simulink model "gm_uz_ssi_interface_2023a"  (R2023a)
settings: Solver=FixedStepDiscrete  StartTime=0.0  StopTime=0.0025  RelTol=1e-3
undefined symbols (not defined in the file or in its folder): binary_or_gray, bit_sum, delay_first_clk_on_off, f_ADC, f_clock, PLL, ssi_clk_divider, ssi_encoder_bit_width_multi_turn, ssi_encoder_bit_width_single_turn, ssi_encoder_number_of_status_bits, t_ADC, t_clock
libraries: hdlmdlgenlib x111, hdlsllib x62, simulink x27, simulink_extras x7
(part 2 of 4)

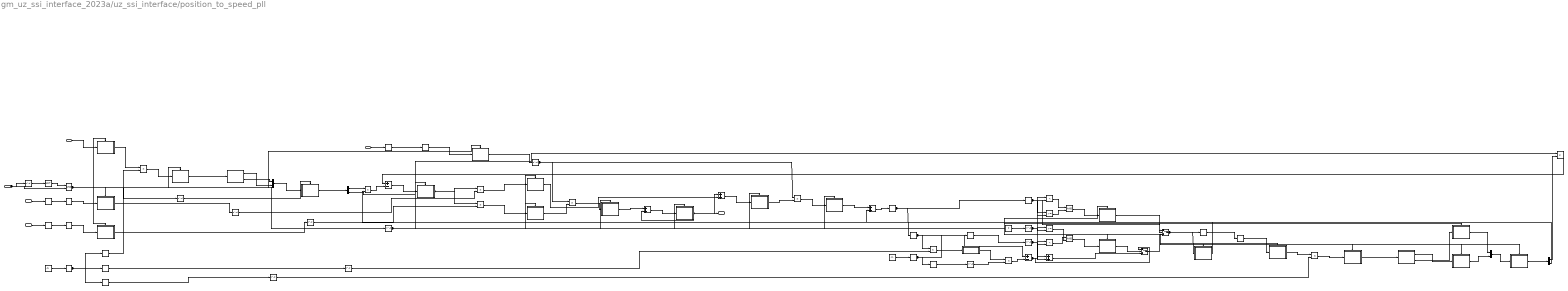
== system gm_uz_ssi_interface_2023a/uz_ssi_interface/position_to_speed_pll ==
  note: pi_controller
  note: +/- 198000
  note: -2 ... 2
  note: wrap 2pi
  note: <<1
  note: phase discriminator
  note: -1 ... 1
  note: pll
  note: -1 ... 1
  note: integrator
  note: 20
  note: +/- 1300
  note: remainder
  position_mech_SI : Inport  OutDataTypeStr=fixdt(0, 27, 24)  PortDimensions=1  SampleTime=1e-08
  t_sample : Inport  Port=2  OutDataTypeStr=fixdt(0, 18, 24)  PortDimensions=1  SampleTime=1e-08
  kp_pll : Inport  Port=3  OutDataTypeStr=fixdt(0, 18, 5)  PortDimensions=1  SampleTime=1e-08
  ki_pll : Inport  Port=4  OutDataTypeStr=fixdt(0, 18, 0)  PortDimensions=1  SampleTime=1e-08
  Trigger : Inport  Port=5  OutDataTypeStr=boolean  SampleTime=1e-08
  AND : Logic  AllPortsSameDT=off  OutDataTypeStr=boolean  SampleTime=1e-08
  AND1 : Logic  AllPortsSameDT=off  OutDataTypeStr=boolean  SampleTime=1e-08
  Constant1 : Constant  Value=0.1591548919677734375  OutDataTypeStr=fixdt(0, 18, 20)  SampleTime=1e-08
  Constant7 : Constant  Value=0  OutDataTypeStr=fixdt(0, 27, 24)  SampleTime=1e-08
  Constant8 : Constant  Value=6.283172607421875  OutDataTypeStr=fixdt(0, 18, 15)  SampleTime=1e-08
  Delay : Subsystem
      settings: MinAlgLoopOccurrences=on
  Delay1 : Subsystem
      settings: MinAlgLoopOccurrences=on
  Delay10 : Subsystem
      settings: MinAlgLoopOccurrences=on
  Delay11 : Subsystem
      settings: MinAlgLoopOccurrences=on
  Delay12 : Subsystem
      settings: MinAlgLoopOccurrences=on
  Delay13 : Subsystem
      settings: MinAlgLoopOccurrences=on
  Delay14 : Subsystem
      settings: MinAlgLoopOccurrences=on
  Delay18 : Subsystem
      settings: MinAlgLoopOccurrences=on
  Delay19 : Subsystem
      settings: MinAlgLoopOccurrences=on
  Delay2 : Subsystem
      settings: MinAlgLoopOccurrences=on
  Delay20 : Subsystem
      settings: MinAlgLoopOccurrences=on
  Delay21 : Subsystem
      settings: MinAlgLoopOccurrences=on
  Delay22 : Subsystem
      settings: MinAlgLoopOccurrences=on
  Delay23 : Subsystem
      settings: MinAlgLoopOccurrences=on
  Delay3 : Subsystem
      settings: MinAlgLoopOccurrences=on
  Delay4 : Subsystem
      settings: MinAlgLoopOccurrences=on
  Delay5 : Subsystem
      settings: MinAlgLoopOccurrences=on
  Delay6 : Subsystem
      settings: MinAlgLoopOccurrences=on
  Delay7 : Subsystem
      settings: MinAlgLoopOccurrences=on
  Delay8 : Subsystem
      settings: MinAlgLoopOccurrences=on
  Delay9 : Subsystem
      settings: MinAlgLoopOccurrences=on
  From{,1..6,11,13..15} (11 alike) : hdlmdlgenlib/Buffer
  Goto{,1..3,8,10..11} (7 alike) : hdlmdlgenlib/Buffer
  Product1 : Product  Inputs=**  OutDataTypeStr=fixdt(1, 27, 23)  SampleTime=1e-08
  Product10 : Product  Inputs=**  OutDataTypeStr=fixdt(1, 27, 20)  SampleTime=1e-08
  Product2 : Product  Inputs=**  OutDataTypeStr=fixdt(1, 27, 25)  SampleTime=1e-08
  Product3 : Product  Inputs=**  OutDataTypeStr=fixdt(1, 27, 25)  SampleTime=1e-08
  Product4 : Product  Inputs=**  OutDataTypeStr=fixdt(1, 27, 20)  SampleTime=1e-08
  Product5 : Product  Inputs=**  OutDataTypeStr=fixdt(1, 27, 8)  SampleTime=1e-08
  Product6 : Product  Inputs=**  OutDataTypeStr=fixdt(1, 27, 14)  SampleTime=1e-08
  Product7 : Product  Inputs=**  OutDataTypeStr=fixdt(1, 27, 23)  SampleTime=1e-08
  Product8 : Product  Inputs=**  OutDataTypeStr=fixdt(1, 27, 26)  SampleTime=1e-08
  Product9 : Product  Inputs=**  OutDataTypeStr=fixdt(1, 27, 20)  SampleTime=1e-08
  Relational Operator1 : RelationalOperator  Operator=<  OutDataTypeStr=boolean  SampleTime=1e-08  InputSameDT=off
  Relational Operator2 : RelationalOperator  OutDataTypeStr=boolean  SampleTime=1e-08  InputSameDT=off
  Relational Operator3 : RelationalOperator  Operator=<  OutDataTypeStr=boolean  SampleTime=1e-08  InputSameDT=off
  Relational Operator4 : RelationalOperator  OutDataTypeStr=boolean  SampleTime=1e-08  InputSameDT=off
  Sine HDL Optimized : Subsystem  mask(Sine and Cosine HDL optimized block){OutputFormula=sin(2*pi*u) and cos(2*pi*u), NumDataPoints=double(256), TableDataTypeStr=fixdt(0,26,20), SimulateLUTROMDelay=off}
      mask prompts: OutputFormula "Simulink:masks:OutputFormula_MP"; NumDataPoints "HDLShared:hdlshared:CosineHDL_Npts"; TableDataTypeStr "Simulink:blkprm_prompts:TABLE_UNIFIEDDATATYPE"; SimulateLUTROMDelay "HDLShared:hdlshared:CosineHDL_SimulateLUTDelay"
      mask help: Sine and Cosine HDL optimized block using quarter wave symmetry, and HDL friendly settings.
      mask Help: helpview([docroot '/hdlcoder/helptargets.map'],'SineAndCosineHDL_Optimized');
      mask TypeOptions OutputFormula: sin(2*pi*u) | cos(2*pi*u) | exp(j*2*pi*u) | sin(2*pi*u) and cos(2*pi*u)
      mask Display:
      | port_label('input',1,'u')
      | port_label('output',1,'sin(2*pi*u)')
      | port_label('output',2,'cos(2*pi*u)')
      | xpos = 0.35;
      | yoffset = 0.5;
      | if ( SimulateLUTROMDelay )
      |   text(xpos,yoffset,'HDL (Z^{-1})','texmode','on')
      | else
      |    text(xpos,yoffset,'HDL')
      | end
  Sine HDL Optimized1 : Subsystem  mask(Sine and Cosine HDL optimized block){OutputFormula=sin(2*pi*u) and cos(2*pi*u), NumDataPoints=double(256), TableDataTypeStr=fixdt(0,26,20), SimulateLUTROMDelay=off}
      mask prompts: OutputFormula "Simulink:masks:OutputFormula_MP"; NumDataPoints "HDLShared:hdlshared:CosineHDL_Npts"; TableDataTypeStr "Simulink:blkprm_prompts:TABLE_UNIFIEDDATATYPE"; SimulateLUTROMDelay "HDLShared:hdlshared:CosineHDL_SimulateLUTDelay"
      mask help: Sine and Cosine HDL optimized block using quarter wave symmetry, and HDL friendly settings.
      mask Help: helpview([docroot '/hdlcoder/helptargets.map'],'SineAndCosineHDL_Optimized');
      mask TypeOptions OutputFormula: sin(2*pi*u) | cos(2*pi*u) | exp(j*2*pi*u) | sin(2*pi*u) and cos(2*pi*u)
      mask Display:
      | port_label('input',1,'u')
      | port_label('output',1,'sin(2*pi*u)')
      | port_label('output',2,'cos(2*pi*u)')
      | xpos = 0.35;
      | yoffset = 0.5;
      | if ( SimulateLUTROMDelay )
      |   text(xpos,yoffset,'HDL (Z^{-1})','texmode','on')
      | else
      |    text(xpos,yoffset,'HDL')
      | end
  Sum1 : Sum  Inputs=+-  AccumDataTypeStr=fixdt(1, 27, 24)  OutDataTypeStr=fixdt(1, 27, 24)  SampleTime=1e-08
  Sum2 : Sum  AccumDataTypeStr=fixdt(1, 32, 20)  OutDataTypeStr=fixdt(1, 27, 16)  SampleTime=1e-08
  Sum3 : Sum  AccumDataTypeStr=fixdt(1, 30, 16)  OutDataTypeStr=fixdt(1, 27, 14)  SampleTime=1e-08
  Sum4 : Sum  AccumDataTypeStr=fixdt(1, 31, 26)  OutDataTypeStr=fixdt(1, 27, 23)  SampleTime=1e-08
  Sum5 : Sum  Inputs=+-  AccumDataTypeStr=fixdt(1, 28, 23)  OutDataTypeStr=fixdt(1, 27, 23)  SampleTime=1e-08
  Sum6 : Sum  AccumDataTypeStr=fixdt(1, 28, 23)  OutDataTypeStr=fixdt(1, 27, 23)  SampleTime=1e-08
  Switch3 : Switch  Criteria=u2 > Threshold  Threshold=double(0)  OutDataTypeStr=fixdt(1, 27, 23)  SampleTime=1e-08  SaturateOnIntegerOverflow=off  InputSameDT=off
  Switch4 : Switch  Criteria=u2 > Threshold  Threshold=double(0)  OutDataTypeStr=fixdt(1, 27, 23)  SampleTime=1e-08  SaturateOnIntegerOverflow=off  InputSameDT=off
  Trigger_delay : Delay  DelayLength=double(1)  InitialCondition=0
  Trigger_delayed_inverted_and_Trigger : Logic  AllPortsSameDT=off  OutDataTypeStr=boolean  SampleTime=1e-08
  delayMatch{,1..9} (10 alike) : Delay  DelayLength=double(1)  InitialCondition=0
  fixed_point_floor : Subsystem
  mux : Mux  Inputs=2
  mux1 : Mux  Inputs=2
  not_Trigger_delayed : Logic  Operator=NOT  Inputs=1  AllPortsSameDT=off  OutDataTypeStr=boolean  SampleTime=1e-08
  t : Demux  Outputs=2
  t1 : Demux  Outputs=2
  speed_mech_SI : Outport  SampleTime=1e-08  InitialOutput=0
  wires:
  Trigger_delay/1 -> not_Trigger_delayed/1
  not_Trigger_delayed/1 -> Trigger_delayed_inverted_and_Trigger/1
  delayMatch/1 -> Delay1/Enable
  mux/1 -> Delay1/1(in0)
  Sine HDL Optimized1/1(x) -> mux/2
  Sine HDL Optimized1/2(y) -> mux/1
  Constant1/1 -> Goto3/1
  delayMatch3/1 -> Relational Operator4/2, Relational Operator2/2
  Constant8/1 -> Goto11/1
  Delay1/1(out0) -> t/1
  Delay13/1(out0) -> Product10/1
  Delay14/1(out0) -> Sine HDL Optimized1/1(u)
  delayMatch7/1 -> Product8/1, Product4/1
  delayMatch9/1 -> Product5/2
  delayMatch6/1 -> Product6/2
  From/1 -> Delay6/1(in0)
  From1/1 -> Delay8/1(in0)
  delayMatch2/1 -> Sum6/2, Relational Operator3/2, Relational Operator1/2
  delayMatch5/1 -> Product1/2
  From2/1 -> Delay7/1(in0)
  delayMatch4/1 -> Product7/2
  delayMatch8/1 -> Product9/2
  From6/1 -> Product10/2
  Goto/1 -> From/1
  Goto1/1 -> From1/1
  Goto11/1 -> From14/1, From13/1
  Goto2/1 -> From2/1
  Goto3/1 -> From6/1, From5/1, From4/1
  Product10/1 -> Delay14/1(in0)
  t/1 -> Product2/1
  t/2 -> Product3/1
  position_mech_SI/1 -> Delay13/1(in0)
  t_sample/1 -> Goto/1
  kp_pll/1 -> Goto1/1
  ki_pll/1 -> Goto2/1
  Trigger/1 -> Trigger_delayed_inverted_and_Trigger/2, Trigger_delay/1
  delayMatch1/1 -> Delay9/Enable, Delay5/Enable, Delay4/Enable, Delay3/Enable, Delay23/Enable, Delay22/Enable, Delay21/Enable, Delay20/Enable, Delay2/Enable, Delay19/Enable, Delay18/Enable, Delay12/Enable, Delay11/Enable, Delay10/Enable, Delay/Enable
  Trigger_delayed_inverted_and_Trigger/1 -> delayMatch1/1, delayMatch/1, Delay8/Enable, Delay7/Enable, Delay6/Enable, Delay14/Enable, Delay13/Enable
  From13/1 -> delayMatch2/1
  Constant7/1 -> delayMatch3/1
  From4/1 -> delayMatch4/1
  From14/1 -> delayMatch5/1
  Delay8/1(out0) -> delayMatch6/1
  Delay6/1(out0) -> delayMatch7/1
  From5/1 -> delayMatch8/1
  Delay7/1(out0) -> delayMatch9/1
  Product2/1 -> Sum1/2
  Delay22/1(out0) -> mux1/2
  Sum6/1 -> Switch4/3
  Relational Operator4/1 -> AND1/2
  Relational Operator3/1 -> AND1/1
  AND1/1 -> Delay20/1(in0)
  Delay20/1(out0) -> Switch4/2
  Product7/1 -> fixed_point_floor/1(x)
  fixed_point_floor/1(y) -> Product1/1
  Product1/1 -> Sum5/2
  From15/1 -> Sum5/1, Product7/1
  Sum5/1 -> Switch4/1, Sum6/1, Relational Operator4/1, Relational Operator3/1
  Switch4/1 -> Switch3/3
  Relational Operator2/1 -> AND/2
  Relational Operator1/1 -> AND/1
  AND/1 -> Delay21/1(in0)
  Delay21/1(out0) -> Switch3/2
  Delay19/1(out0) -> Sum4/2
  Product6/1 -> Delay3/1(in0)
  Delay3/1(out0) -> Sum3/2
  Sum3/1 -> Delay9/1(in0)
  Delay9/1(out0) -> Product8/2
  Product8/1 -> Delay10/1(in0)
  Delay10/1(out0) -> Sum4/1
  Sum4/1 -> Goto10/1
  Goto10/1 -> From15/1, From11/1
  From11/1 -> Switch3/1, Relational Operator2/1, Relational Operator1/1
  Switch3/1 -> Delay19/1(in0), Goto8/1
  Goto8/1 -> From3/1
  From3/1 -> Delay11/1(in0)
  Delay11/1(out0) -> Product9/1
  Product9/1 -> Delay12/1(in0)
  Delay12/1(out0) -> Sine HDL Optimized/1(u)
  Sine HDL Optimized/1(x) -> Delay22/1(in0)
  Sine HDL Optimized/2(y) -> Delay23/1(in0)
  Delay23/1(out0) -> mux1/1
  mux1/1 -> Delay18/1(in0)
  Delay18/1(out0) -> t1/1
  t1/1 -> Product3/2
  t1/2 -> Product2/2
  Product3/1 -> Sum1/1
  Sum1/1 -> Delay2/1(in0)
  Delay2/1(out0) -> Product6/1, Product5/1
  Product5/1 -> Delay5/1(in0)
  Delay5/1(out0) -> Product4/2
  Product4/1 -> Delay4/1(in0)
  Delay4/1(out0) -> Sum2/1
  Sum2/1 -> Delay/1(in0)
  Delay/1(out0) -> Sum3/1, Sum2/2, speed_mech_SI/1

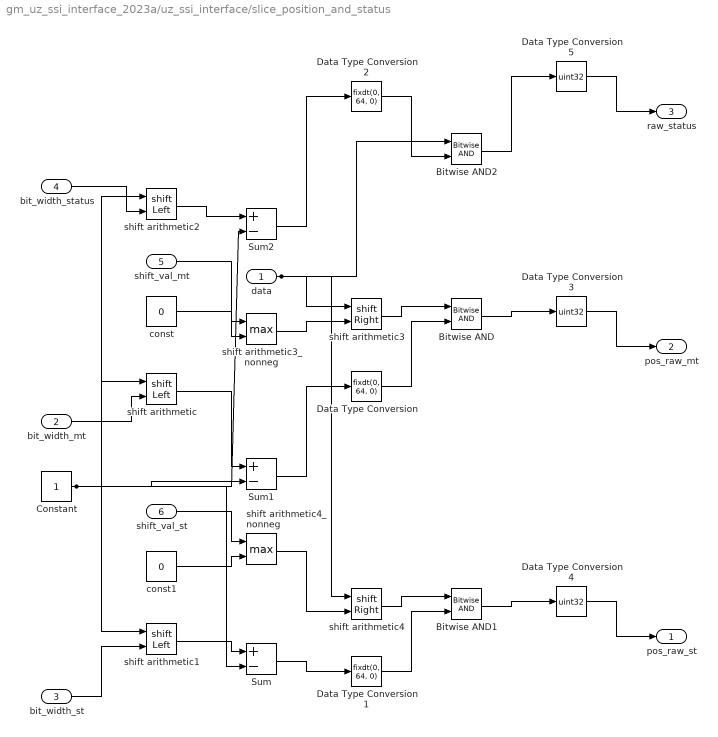
== system gm_uz_ssi_interface_2023a/uz_ssi_interface/slice_position_and_status ==
  data : Inport  OutDataTypeStr=fixdt(0, 64, 0)  PortDimensions=1  SampleTime=1e-08
  bit_width_mt : Inport  Port=2  OutDataTypeStr=uint32  PortDimensions=1  SampleTime=1e-08
  bit_width_st : Inport  Port=3  OutDataTypeStr=uint32  PortDimensions=1  SampleTime=1e-08
  bit_width_status : Inport  Port=4  OutDataTypeStr=uint32  PortDimensions=1  SampleTime=1e-08
  shift_val_mt : Inport  Port=5  OutDataTypeStr=int32  PortDimensions=1  SampleTime=1e-08
  shift_val_st : Inport  Port=6  OutDataTypeStr=int32  PortDimensions=1  SampleTime=1e-08
  Bitwise AND : simulink/Logic and Bit Operations/Bitwise Operator  logicop=AND  UseBitMask=off  NumInputPorts=2  BitMask=double(0)  BitMaskRealWorld=Real World Value
  Bitwise AND1 : simulink/Logic and Bit Operations/Bitwise Operator  logicop=AND  UseBitMask=off  NumInputPorts=2  BitMask=double(0)  BitMaskRealWorld=Real World Value
  Bitwise AND2 : simulink/Logic and Bit Operations/Bitwise Operator  logicop=AND  UseBitMask=off  NumInputPorts=2  BitMask=double(0)  BitMaskRealWorld=Real World Value
  Constant : Constant  OutDataTypeStr=uint32  SampleTime=1e-08
  Data Type Conversion : DataTypeConversion  OutDataTypeStr=fixdt(0, 64, 0)  SampleTime=1e-08  SaturateOnIntegerOverflow=off  RndMeth=Floor
  Data Type Conversion1 : DataTypeConversion  OutDataTypeStr=fixdt(0, 64, 0)  SampleTime=1e-08  SaturateOnIntegerOverflow=off  RndMeth=Floor
  Data Type Conversion2 : DataTypeConversion  OutDataTypeStr=fixdt(0, 64, 0)  SampleTime=1e-08  SaturateOnIntegerOverflow=off  RndMeth=Floor
  Data Type Conversion3 : DataTypeConversion  OutDataTypeStr=uint32  SampleTime=1e-08  SaturateOnIntegerOverflow=off  RndMeth=Floor
  Data Type Conversion4 : DataTypeConversion  OutDataTypeStr=uint32  SampleTime=1e-08  SaturateOnIntegerOverflow=off  RndMeth=Floor
  Data Type Conversion5 : DataTypeConversion  OutDataTypeStr=uint32  SampleTime=1e-08  SaturateOnIntegerOverflow=off  RndMeth=Floor
  Sum : Sum  Inputs=+-  AccumDataTypeStr=uint32  OutDataTypeStr=uint32  SampleTime=1e-08
  Sum1 : Sum  Inputs=+-  AccumDataTypeStr=uint32  OutDataTypeStr=uint32  SampleTime=1e-08
  Sum2 : Sum  Inputs=+-  AccumDataTypeStr=uint32  OutDataTypeStr=uint32  SampleTime=1e-08
  const : Constant  Value=0  OutDataTypeStr=int32  SampleTime=1e-08
  const1 : Constant  Value=0  OutDataTypeStr=int32  SampleTime=1e-08
  shift arithmetic : ArithShift  BitShiftNumberSource=Input port  BitShiftDirection=Left
      settings: InputPortMap=u0,p1
  shift arithmetic1 : ArithShift  BitShiftNumberSource=Input port  BitShiftDirection=Left
      settings: InputPortMap=u0,p1
  shift arithmetic2 : ArithShift  BitShiftNumberSource=Input port  BitShiftDirection=Left
      settings: InputPortMap=u0,p1
  shift arithmetic3 : ArithShift  BitShiftNumberSource=Input port  BitShiftDirection=Right
      settings: InputPortMap=u0,p1
  shift arithmetic3_nonneg : MinMax  Function=max  Inputs=2
  shift arithmetic4 : ArithShift  BitShiftNumberSource=Input port  BitShiftDirection=Right
      settings: InputPortMap=u0,p1
  shift arithmetic4_nonneg : MinMax  Function=max  Inputs=2
  pos_raw_st : Outport  SampleTime=1e-08
  pos_raw_mt : Outport  Port=2  SampleTime=1e-08
  raw_status : Outport  Port=3  SampleTime=1e-08
  wires:
  Bitwise AND/1 -> Data Type Conversion3/1
  Bitwise AND1/1 -> Data Type Conversion4/1
  Bitwise AND2/1 -> Data Type Conversion5/1
  Constant/1 -> Sum2/2, Sum1/2, Sum/2, shift arithmetic2/1, shift arithmetic1/1, shift arithmetic/1
  Data Type Conversion/1 -> Bitwise AND/2
  Data Type Conversion1/1 -> Bitwise AND1/2
  Data Type Conversion2/1 -> Bitwise AND2/2
  Data Type Conversion3/1 -> pos_raw_mt/1
  Data Type Conversion4/1 -> pos_raw_st/1
  Data Type Conversion5/1 -> raw_status/1
  shift arithmetic/1 -> Sum1/1
  shift arithmetic1/1 -> Sum/1
  shift arithmetic2/1 -> Sum2/1
  shift arithmetic3/1 -> Bitwise AND/1
  shift arithmetic4/1 -> Bitwise AND1/1
  Sum/1 -> Data Type Conversion1/1
  Sum1/1 -> Data Type Conversion/1
  Sum2/1 -> Data Type Conversion2/1
  shift arithmetic3_nonneg/1 -> shift arithmetic3/2
  const/1 -> shift arithmetic3_nonneg/2
  shift arithmetic4_nonneg/1 -> shift arithmetic4/2
  const1/1 -> shift arithmetic4_nonneg/2
  data/1 -> shift arithmetic4/1, shift arithmetic3/1, Bitwise AND2/1
  bit_width_mt/1 -> shift arithmetic/2
  bit_width_st/1 -> shift arithmetic1/2
  bit_width_status/1 -> shift arithmetic2/2
  shift_val_mt/1 -> shift arithmetic3_nonneg/1
  shift_val_st/1 -> shift arithmetic4_nonneg/1

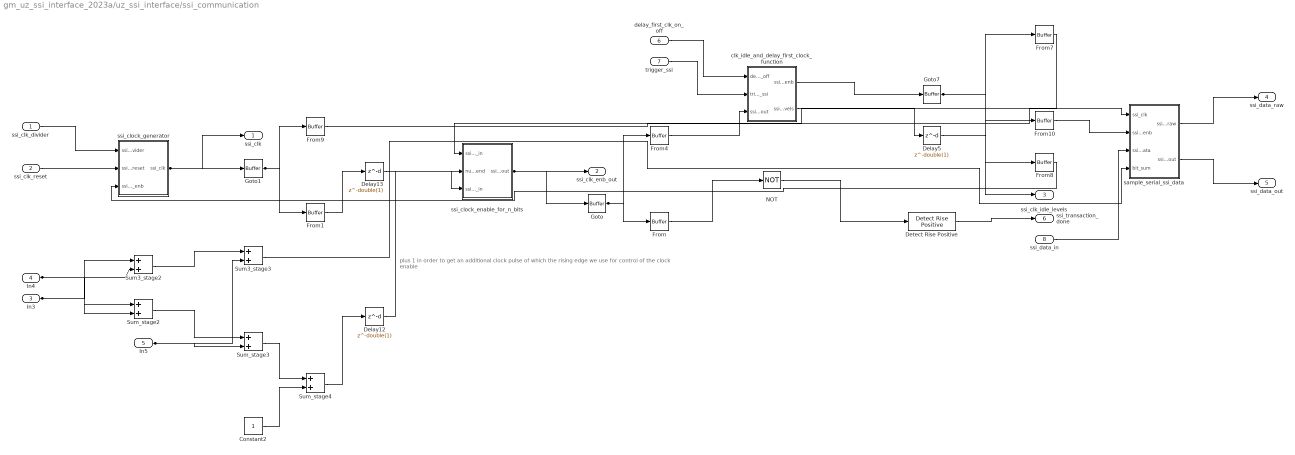
== system gm_uz_ssi_interface_2023a/uz_ssi_interface/ssi_communication ==
  note: plus 1 in order to get an additional clock pulse of which the rising edge we use for control of the clock enable
  ssi_clk_divider : Inport  OutDataTypeStr=uint32  PortDimensions=1  SampleTime=1e-08
  ssi_clk_reset : Inport  Port=2  OutDataTypeStr=boolean  PortDimensions=1  SampleTime=1e-08
  In3 : Inport  Port=3  OutDataTypeStr=uint32  PortDimensions=1  SampleTime=1e-08
  In4 : Inport  Port=4  OutDataTypeStr=uint32  PortDimensions=1  SampleTime=1e-08
  In5 : Inport  Port=5  OutDataTypeStr=uint32  PortDimensions=1  SampleTime=1e-08
  delay_first_clk_on_off : Inport  Port=6  OutDataTypeStr=boolean  PortDimensions=1  SampleTime=1e-08
  trigger_ssi : Inport  Port=7  OutDataTypeStr=boolean  PortDimensions=1  SampleTime=1e-08
  ssi_data_in : Inport  Port=8  OutDataTypeStr=boolean  PortDimensions=1  SampleTime=1e-08
  Constant2 : Constant  OutDataTypeStr=uint32  SampleTime=1e-08
  Delay12 : Delay  DelayLength=double(1)  InitialCondition=0  SampleTime=1e-08
  Delay13 : Delay  DelayLength=double(1)  InitialCondition=0  SampleTime=1e-08
  Delay5 : Delay  DelayLength=double(1)  InitialCondition=0  SampleTime=1e-08
  Detect Rise Positive : simulink/Logic and Bit Operations/Detect Rise Positive  vinit=0  OutDataTypeStr=boolean
  From{,1,4,7..10} (7 alike) : hdlmdlgenlib/Buffer
  Goto : hdlmdlgenlib/Buffer
  Goto1 : hdlmdlgenlib/Buffer
  Goto7 : hdlmdlgenlib/Buffer
  NOT : Logic  Operator=NOT  Inputs=1  AllPortsSameDT=off  OutDataTypeStr=boolean  SampleTime=1e-08
  Sum3_stage2 : Sum  AccumDataTypeStr=uint32  OutDataTypeStr=fixdt(0, 33, 0)  SampleTime=1e-08
  Sum3_stage3 : Sum  AccumDataTypeStr=uint32  OutDataTypeStr=uint32  SampleTime=1e-08
  Sum_stage2 : Sum  AccumDataTypeStr=uint32  OutDataTypeStr=fixdt(0, 33, 0)  SampleTime=1e-08
  Sum_stage3 : Sum  AccumDataTypeStr=uint32  OutDataTypeStr=fixdt(0, 34, 0)  SampleTime=1e-08
  Sum_stage4 : Sum  AccumDataTypeStr=uint32  OutDataTypeStr=uint32  SampleTime=1e-08
  clk_idle_and_delay_first_clock_function : Subsystem
  sample_serial_ssi_data : Subsystem
  ssi_clock_enable_for_n_bits : Subsystem
  ssi_clock_generator : Subsystem
  ssi_clk : Outport  SampleTime=1e-08
  ssi_clk_enb_out : Outport  Port=2  SampleTime=1e-08
  ssi_clk_idle_levels : Outport  Port=3  SampleTime=1e-08
  ssi_data_raw : Outport  Port=4  SampleTime=1e-08
  ssi_data_out : Outport  Port=5  SampleTime=1e-08
  ssi_transaction_done : Outport  Port=6  SampleTime=1e-08
  wires:
  Constant2/1 -> Sum_stage4/2
  Delay12/1 -> ssi_clock_enable_for_n_bits/2(num_of_clock_pulses_to_send)
  Delay5/1 -> ssi_clk_idle_levels/1
  Detect Rise Positive/1 -> ssi_transaction_done/1
  From/1 -> NOT/1
  From10/1 -> sample_serial_ssi_data/2(ssi_clk_enb)
  From9/1 -> sample_serial_ssi_data/1(ssi_clk)
  NOT/1 -> Detect Rise Positive/1
  Sum_stage4/1 -> Delay12/1
  Sum3_stage3/1 -> sample_serial_ssi_data/4(bit_sum)
  clk_idle_and_delay_first_clock_function/2(ssi_clk_idle_levels) -> Delay5/1
  sample_serial_ssi_data/1(ssi_data_raw) -> ssi_data_raw/1
  sample_serial_ssi_data/2(ssi_data_out) -> ssi_data_out/1
  ssi_clock_enable_for_n_bits/1(ssi_clk_enb_out) -> ssi_clk_enb_out/1, Goto/1
  ssi_clock_generator/1(ssi_clk) -> ssi_clk/1, Goto1/1
  Goto/1 -> From/1, From4/1
  Goto1/1 -> From9/1, From1/1
  Goto7/1 -> From10/1, From7/1, From8/1
  Sum_stage2/1 -> Sum_stage3/1
  Sum_stage3/1 -> Sum_stage4/1
  Sum3_stage2/1 -> Sum3_stage3/1
  ssi_clk_divider/1 -> ssi_clock_generator/1(ssi_clk_divider)
  ssi_clk_reset/1 -> ssi_clock_generator/2(ssi_clk_reset)
  In3/1 -> Sum3_stage2/1, Sum_stage2/1
  In4/1 -> Sum3_stage2/2, Sum_stage2/2
  In5/1 -> Sum3_stage3/2, Sum_stage3/2
  delay_first_clk_on_off/1 -> clk_idle_and_delay_first_clock_function/1(delay_first_clk_on_off)
  trigger_ssi/1 -> clk_idle_and_delay_first_clock_function/2(trigger_ssi)
  ssi_data_in/1 -> sample_serial_ssi_data/3(ssi_data)
  Delay13/1 -> ssi_clock_enable_for_n_bits/3(ssi_clk_in)
  clk_idle_and_delay_first_clock_function/1(ssi_clk_enb) -> Goto7/1
  From4/1 -> clk_idle_and_delay_first_clock_function/3(ssi_clk_enb_out)
  From1/1 -> Delay13/1
  From8/1 -> ssi_clock_generator/3(ssi_clk_enb)
  From7/1 -> ssi_clock_enable_for_n_bits/1(ssi_clk_enb_in)

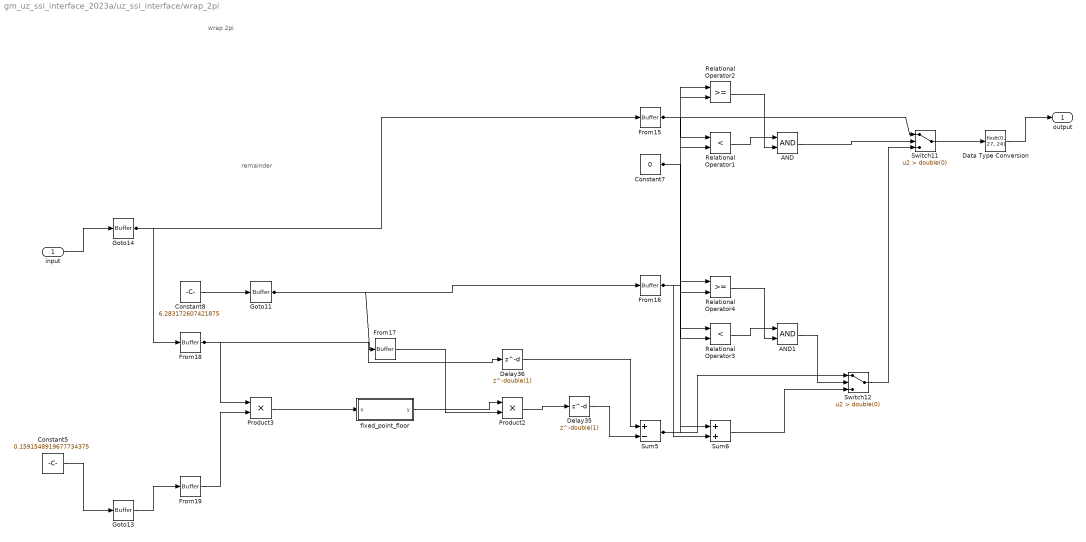
== system gm_uz_ssi_interface_2023a/uz_ssi_interface/wrap_2pi ==
  note: remainder
  note: wrap 2pi
  input : Inport  OutDataTypeStr=fixdt(0, 27, 20)  PortDimensions=1  SampleTime=1e-08
  AND : Logic  AllPortsSameDT=off  OutDataTypeStr=boolean  SampleTime=1e-08
  AND1 : Logic  AllPortsSameDT=off  OutDataTypeStr=boolean  SampleTime=1e-08
  Constant5 : Constant  Value=0.1591548919677734375  OutDataTypeStr=fixdt(0, 18, 20)  SampleTime=1e-08
  Constant7 : Constant  Value=0  OutDataTypeStr=fixdt(0, 27, 24)  SampleTime=1e-08
  Constant8 : Constant  Value=6.283172607421875  OutDataTypeStr=fixdt(0, 18, 15)  SampleTime=1e-08
  Data Type Conversion : DataTypeConversion  OutDataTypeStr=fixdt(0, 27, 24)  SampleTime=1e-08  SaturateOnIntegerOverflow=off  RndMeth=Floor
  Delay35 : Delay  DelayLength=double(1)  InitialCondition=0  SampleTime=1e-08
  Delay36 : Delay  DelayLength=double(1)  InitialCondition=0  SampleTime=1e-08
  From{15..19} (5 alike) : hdlmdlgenlib/Buffer
  Goto11 : hdlmdlgenlib/Buffer
  Goto13 : hdlmdlgenlib/Buffer
  Goto14 : hdlmdlgenlib/Buffer
  Product2 : Product  Inputs=**  OutDataTypeStr=fixdt(0, 27, 24)  SampleTime=1e-08
  Product3 : Product  Inputs=**  OutDataTypeStr=fixdt(0, 27, 24)  SampleTime=1e-08
  Relational Operator1 : RelationalOperator  Operator=<  OutDataTypeStr=boolean  SampleTime=1e-08  InputSameDT=off
  Relational Operator2 : RelationalOperator  OutDataTypeStr=boolean  SampleTime=1e-08  InputSameDT=off
  Relational Operator3 : RelationalOperator  Operator=<  OutDataTypeStr=boolean  SampleTime=1e-08  InputSameDT=off
  Relational Operator4 : RelationalOperator  OutDataTypeStr=boolean  SampleTime=1e-08  InputSameDT=off
  Sum5 : Sum  Inputs=+-  AccumDataTypeStr=fixdt(1, 32, 24)  OutDataTypeStr=fixdt(0, 27, 24)  SampleTime=1e-08
  Sum6 : Sum  AccumDataTypeStr=fixdt(0, 28, 24)  OutDataTypeStr=fixdt(0, 27, 24)  SampleTime=1e-08
  Switch11 : Switch  Criteria=u2 > Threshold  Threshold=double(0)  OutDataTypeStr=fixdt(0, 27, 20)  SampleTime=1e-08  SaturateOnIntegerOverflow=off  InputSameDT=off
  Switch12 : Switch  Criteria=u2 > Threshold  Threshold=double(0)  OutDataTypeStr=fixdt(0, 27, 24)  SampleTime=1e-08  SaturateOnIntegerOverflow=off  InputSameDT=off
  fixed_point_floor : Subsystem
  output : Outport  SampleTime=1e-08
  wires:
  AND/1 -> Switch11/2
  AND1/1 -> Switch12/2
  Constant5/1 -> Goto13/1
  Constant7/1 -> Relational Operator4/2, Relational Operator2/2
  Constant8/1 -> Goto11/1
  Data Type Conversion/1 -> output/1
  Delay35/1 -> Sum5/2
  Delay36/1 -> Sum5/1
  From15/1 -> Switch11/1, Relational Operator2/1, Relational Operator1/1
  From16/1 -> Sum6/2, Relational Operator3/2, Relational Operator1/2
  From17/1 -> Product2/2
  From18/1 -> Product3/1, Delay36/1
  From19/1 -> Product3/2
  Product2/1 -> Delay35/1
  Product3/1 -> fixed_point_floor/1(x)
  Relational Operator1/1 -> AND/1
  Relational Operator2/1 -> AND/2
  Relational Operator3/1 -> AND1/1
  Relational Operator4/1 -> AND1/2
  Sum5/1 -> Switch12/1, Sum6/1, Relational Operator4/1, Relational Operator3/1
  Sum6/1 -> Switch12/3
  Switch11/1 -> Data Type Conversion/1
  Switch12/1 -> Switch11/3
  fixed_point_floor/1(y) -> Product2/1
  Goto14/1 -> From18/1, From15/1
  Goto11/1 -> From17/1, From16/1
  Goto13/1 -> From19/1
  input/1 -> Goto14/1

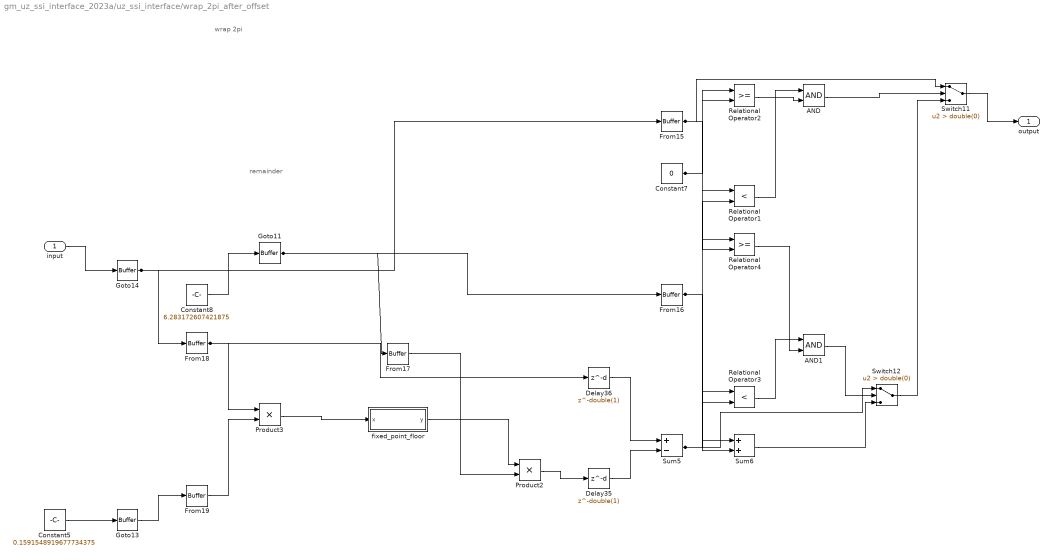
== system gm_uz_ssi_interface_2023a/uz_ssi_interface/wrap_2pi_after_offset ==
  note: remainder
  note: wrap 2pi
  input : Inport  OutDataTypeStr=fixdt(1, 27, 23)  PortDimensions=1  SampleTime=1e-08
  AND : Logic  AllPortsSameDT=off  OutDataTypeStr=boolean  SampleTime=1e-08
  AND1 : Logic  AllPortsSameDT=off  OutDataTypeStr=boolean  SampleTime=1e-08
  Constant5 : Constant  Value=0.1591548919677734375  OutDataTypeStr=fixdt(0, 18, 20)  SampleTime=1e-08
  Constant7 : Constant  Value=0  OutDataTypeStr=fixdt(0, 27, 24)  SampleTime=1e-08
  Constant8 : Constant  Value=6.283172607421875  OutDataTypeStr=fixdt(0, 18, 15)  SampleTime=1e-08
  Delay35 : Delay  DelayLength=double(1)  InitialCondition=0  SampleTime=1e-08
  Delay36 : Delay  DelayLength=double(1)  InitialCondition=0  SampleTime=1e-08
  From{15..19} (5 alike) : hdlmdlgenlib/Buffer
  Goto11 : hdlmdlgenlib/Buffer
  Goto13 : hdlmdlgenlib/Buffer
  Goto14 : hdlmdlgenlib/Buffer
  Product2 : Product  Inputs=**  OutDataTypeStr=fixdt(0, 27, 24)  SampleTime=1e-08
  Product3 : Product  Inputs=**  OutDataTypeStr=fixdt(1, 27, 23)  SampleTime=1e-08
  Relational Operator1 : RelationalOperator  Operator=<  OutDataTypeStr=boolean  SampleTime=1e-08  InputSameDT=off
  Relational Operator2 : RelationalOperator  OutDataTypeStr=boolean  SampleTime=1e-08  InputSameDT=off
  Relational Operator3 : RelationalOperator  Operator=<  OutDataTypeStr=boolean  SampleTime=1e-08  InputSameDT=off
  Relational Operator4 : RelationalOperator  OutDataTypeStr=boolean  SampleTime=1e-08  InputSameDT=off
  Sum5 : Sum  Inputs=+-  AccumDataTypeStr=fixdt(1, 29, 24)  OutDataTypeStr=fixdt(0, 27, 24)  SampleTime=1e-08
  Sum6 : Sum  AccumDataTypeStr=fixdt(0, 28, 24)  OutDataTypeStr=fixdt(0, 27, 24)  SampleTime=1e-08
  Switch11 : Switch  Criteria=u2 > Threshold  Threshold=double(0)  OutDataTypeStr=fixdt(0, 27, 24)  SampleTime=1e-08  SaturateOnIntegerOverflow=off  InputSameDT=off
  Switch12 : Switch  Criteria=u2 > Threshold  Threshold=double(0)  OutDataTypeStr=fixdt(0, 27, 24)  SampleTime=1e-08  SaturateOnIntegerOverflow=off  InputSameDT=off
  fixed_point_floor : Subsystem
  output : Outport  SampleTime=1e-08
  wires:
  AND/1 -> Switch11/2
  AND1/1 -> Switch12/2
  Constant5/1 -> Goto13/1
  Constant7/1 -> Relational Operator4/2, Relational Operator2/2
  Constant8/1 -> Goto11/1
  Delay35/1 -> Sum5/2
  Delay36/1 -> Sum5/1
  From15/1 -> Switch11/1, Relational Operator2/1, Relational Operator1/1
  From16/1 -> Sum6/2, Relational Operator3/2, Relational Operator1/2
  From17/1 -> Product2/2
  From18/1 -> Product3/1, Delay36/1
  From19/1 -> Product3/2
  Product2/1 -> Delay35/1
  Product3/1 -> fixed_point_floor/1(x)
  Relational Operator1/1 -> AND/1
  Relational Operator2/1 -> AND/2
  Relational Operator3/1 -> AND1/1
  Relational Operator4/1 -> AND1/2
  Sum5/1 -> Switch12/1, Sum6/1, Relational Operator4/1, Relational Operator3/1
  Sum6/1 -> Switch12/3
  Switch11/1 -> output/1
  Switch12/1 -> Switch11/3
  fixed_point_floor/1(y) -> Product2/1
  Goto14/1 -> From18/1, From15/1
  Goto11/1 -> From17/1, From16/1
  Goto13/1 -> From19/1
  input/1 -> Goto14/1

== system gm_uz_ssi_interface_2023a/uz_ssi_interface/Gray_code_to_binary/gray_to_bin_mt ==
  gray : Inport  OutDataTypeStr=uint32  PortDimensions=1  SampleTime=1e-08
  enb : Inport  Port=2  OutDataTypeStr=boolean  PortDimensions=1  SampleTime=1e-08
  Bitwise OR1 : simulink/Logic and Bit Operations/Bitwise Operator  logicop=XOR  UseBitMask=off  NumInputPorts=2  BitMask=double(0)  BitMaskRealWorld=Real World Value
  Constant4 : Constant  Value=24  OutDataTypeStr=fixdt(0, 6, 0)  SampleTime=1e-08
  Delay : Delay  DelayLength=double(1)  InitialCondition=0  SampleTime=1e-08
  Delay2 : Delay  DelayLength=double(1)  InitialCondition=0  SampleTime=1e-08
  Detect Rise Positive : simulink/Logic and Bit Operations/Detect Rise Positive  vinit=0  OutDataTypeStr=boolean
  Detect Rise Positive1 : simulink/Logic and Bit Operations/Detect Rise Positive  vinit=0  OutDataTypeStr=boolean
  HDL Counter : hdlsllib/Sources/HDL Counter  CountType=Count limited  CountInit=0  CountStep=1  CountMax=24  CountFromType=Initial value  CountFrom=0  CountResetPort=on  CountLoadPort=off  CountEnbPort=on  CountDirPort=off  CountHitOutputPort=off  CountDataType=Unsigned  CountWordLen=6  CountFracLen=0  CountSampTime=t_clock
  OR : Logic  Operator=OR  AllPortsSameDT=off  OutDataTypeStr=boolean  SampleTime=1e-08
  Relational Operator2 : RelationalOperator  Operator===  OutDataTypeStr=boolean  SampleTime=1e-08  InputSameDT=off
  S-R Flip-Flop : simulink_extras/Flip Flops/S-R Flip-Flop  initial_condition=0
  Switch : Switch  Criteria=u2 > Threshold  Threshold=double(0)  OutDataTypeStr=uint32  SampleTime=1e-08  SaturateOnIntegerOverflow=off  InputSameDT=off
  Switch3 : Switch  Criteria=u2 > Threshold  Threshold=double(0)  OutDataTypeStr=uint32  SampleTime=1e-08  SaturateOnIntegerOverflow=off  InputSameDT=off
  shift arithmetic : ArithShift  BitShiftNumberSource=Input port  BitShiftDirection=Right
      settings: InputPortMap=u0,p1
  binary_out : Outport  SampleTime=1e-08
  wires:
  Bitwise OR1/1 -> Delay/1, Switch3/1
  Constant4/1 -> Relational Operator2/2
  Detect Rise Positive/1 -> Switch3/2, S-R Flip-Flop/2
  Detect Rise Positive1/1 -> Switch/2
  HDL Counter/1 -> shift arithmetic/2, Relational Operator2/1
  shift arithmetic/1 -> Bitwise OR1/2
  Switch3/1 -> binary_out/1, Delay2/1
  gray/1 -> shift arithmetic/1, Switch/1
  enb/1 -> Detect Rise Positive1/1, OR/1, S-R Flip-Flop/1
  Delay2/1 -> Switch3/3
  S-R Flip-Flop/1 -> HDL Counter/2
  S-R Flip-Flop/2 -> OR/2
  Relational Operator2/1 -> Detect Rise Positive/1
  OR/1 -> HDL Counter/1
  Delay/1 -> Switch/3
  Switch/1 -> Bitwise OR1/1

== system gm_uz_ssi_interface_2023a/uz_ssi_interface/Gray_code_to_binary/gray_to_bin_st ==
  gray : Inport  OutDataTypeStr=uint32  PortDimensions=1  SampleTime=1e-08
  enb : Inport  Port=2  OutDataTypeStr=boolean  PortDimensions=1  SampleTime=1e-08
  Bitwise OR1 : simulink/Logic and Bit Operations/Bitwise Operator  logicop=XOR  UseBitMask=off  NumInputPorts=2  BitMask=double(0)  BitMaskRealWorld=Real World Value
  Constant4 : Constant  Value=24  OutDataTypeStr=fixdt(0, 6, 0)  SampleTime=1e-08
  Delay : Delay  DelayLength=double(1)  InitialCondition=0  SampleTime=1e-08
  Delay2 : Delay  DelayLength=double(1)  InitialCondition=0  SampleTime=1e-08
  Detect Rise Positive : simulink/Logic and Bit Operations/Detect Rise Positive  vinit=0  OutDataTypeStr=boolean
  Detect Rise Positive1 : simulink/Logic and Bit Operations/Detect Rise Positive  vinit=0  OutDataTypeStr=boolean
  HDL Counter : hdlsllib/Sources/HDL Counter  CountType=Count limited  CountInit=0  CountStep=1  CountMax=24  CountFromType=Initial value  CountFrom=0  CountResetPort=on  CountLoadPort=off  CountEnbPort=on  CountDirPort=off  CountHitOutputPort=off  CountDataType=Unsigned  CountWordLen=6  CountFracLen=0  CountSampTime=t_clock
  OR : Logic  Operator=OR  AllPortsSameDT=off  OutDataTypeStr=boolean  SampleTime=1e-08
  Relational Operator2 : RelationalOperator  Operator===  OutDataTypeStr=boolean  SampleTime=1e-08  InputSameDT=off
  S-R Flip-Flop : simulink_extras/Flip Flops/S-R Flip-Flop  initial_condition=0
  Switch : Switch  Criteria=u2 > Threshold  Threshold=double(0)  OutDataTypeStr=uint32  SampleTime=1e-08  SaturateOnIntegerOverflow=off  InputSameDT=off
  Switch3 : Switch  Criteria=u2 > Threshold  Threshold=double(0)  OutDataTypeStr=uint32  SampleTime=1e-08  SaturateOnIntegerOverflow=off  InputSameDT=off
  shift arithmetic : ArithShift  BitShiftNumberSource=Input port  BitShiftDirection=Right
      settings: InputPortMap=u0,p1
  binary_out : Outport  SampleTime=1e-08
  wires:
  Bitwise OR1/1 -> Delay/1, Switch3/1
  Constant4/1 -> Relational Operator2/2
  Detect Rise Positive/1 -> Switch3/2, S-R Flip-Flop/2
  Detect Rise Positive1/1 -> Switch/2
  HDL Counter/1 -> shift arithmetic/2, Relational Operator2/1
  shift arithmetic/1 -> Bitwise OR1/2
  Switch3/1 -> binary_out/1, Delay2/1
  gray/1 -> shift arithmetic/1, Switch/1
  enb/1 -> Detect Rise Positive1/1, OR/1, S-R Flip-Flop/1
  Delay2/1 -> Switch3/3
  S-R Flip-Flop/1 -> HDL Counter/2
  S-R Flip-Flop/2 -> OR/2
  Relational Operator2/1 -> Detect Rise Positive/1
  OR/1 -> HDL Counter/1
  Delay/1 -> Switch/3
  Switch/1 -> Bitwise OR1/1

== system gm_uz_ssi_interface_2023a/uz_ssi_interface/position_to_speed_pll/Delay ==
  in0 : Inport  OutDataTypeStr=fixdt(1, 27, 16)  SampleTime=1e-08
  Trigger_emulated : EnablePort  OutDataTypeStr=boolean
  Delay : Delay  DelayLength=double(1)  InitialCondition=0
  out0 : Outport  OutDataTypeStr=fixdt(1, 27, 16)  SampleTime=1e-08  InitialOutput=0
  wires:
  Delay/1 -> out0/1
  in0/1 -> Delay/1

== system gm_uz_ssi_interface_2023a/uz_ssi_interface/position_to_speed_pll/Delay1 ==
  in0 : Inport  OutDataTypeStr=fixdt(1, 27, 20)  PortDimensions=[2]  SampleTime=1e-08
  Trigger_emulated : EnablePort  OutDataTypeStr=boolean
  Delay1 : Delay  DelayLength=double(1)  InitialCondition=[1 0]
  out0 : Outport  OutDataTypeStr=fixdt(1, 27, 20)  PortDimensions=[2]  SampleTime=1e-08  InitialOutput=0
  wires:
  Delay1/1 -> out0/1
  in0/1 -> Delay1/1

== system gm_uz_ssi_interface_2023a/uz_ssi_interface/position_to_speed_pll/Delay10 ==
  in0 : Inport  OutDataTypeStr=fixdt(1, 27, 26)  SampleTime=1e-08
  Trigger_emulated : EnablePort  OutDataTypeStr=boolean
  Delay10 : Delay  DelayLength=double(1)  InitialCondition=0
  out0 : Outport  OutDataTypeStr=fixdt(1, 27, 26)  SampleTime=1e-08  InitialOutput=0
  wires:
  Delay10/1 -> out0/1
  in0/1 -> Delay10/1

== system gm_uz_ssi_interface_2023a/uz_ssi_interface/position_to_speed_pll/Delay11 ==
  in0 : Inport  OutDataTypeStr=fixdt(1, 27, 23)  SampleTime=1e-08
  Trigger_emulated : EnablePort  OutDataTypeStr=boolean
  Delay11 : Delay  DelayLength=double(1)  InitialCondition=0
  out0 : Outport  OutDataTypeStr=fixdt(1, 27, 23)  SampleTime=1e-08  InitialOutput=0
  wires:
  Delay11/1 -> out0/1
  in0/1 -> Delay11/1

== system gm_uz_ssi_interface_2023a/uz_ssi_interface/position_to_speed_pll/Delay12 ==
  in0 : Inport  OutDataTypeStr=fixdt(1, 27, 20)  SampleTime=1e-08
  Trigger_emulated : EnablePort  OutDataTypeStr=boolean
  Delay12 : Delay  DelayLength=double(1)  InitialCondition=0
  out0 : Outport  OutDataTypeStr=fixdt(1, 27, 20)  SampleTime=1e-08  InitialOutput=0
  wires:
  Delay12/1 -> out0/1
  in0/1 -> Delay12/1

== system gm_uz_ssi_interface_2023a/uz_ssi_interface/position_to_speed_pll/Delay13 ==
  in0 : Inport  OutDataTypeStr=fixdt(0, 27, 24)  SampleTime=1e-08
  Trigger_emulated : EnablePort  OutDataTypeStr=boolean
  Delay13 : Delay  DelayLength=double(1)  InitialCondition=0
  out0 : Outport  OutDataTypeStr=fixdt(0, 27, 24)  SampleTime=1e-08  InitialOutput=0
  wires:
  Delay13/1 -> out0/1
  in0/1 -> Delay13/1

== system gm_uz_ssi_interface_2023a/uz_ssi_interface/position_to_speed_pll/Delay14 ==
  in0 : Inport  OutDataTypeStr=fixdt(1, 27, 20)  SampleTime=1e-08
  Trigger_emulated : EnablePort  OutDataTypeStr=boolean
  Delay14 : Delay  DelayLength=double(1)  InitialCondition=0
  out0 : Outport  OutDataTypeStr=fixdt(1, 27, 20)  SampleTime=1e-08  InitialOutput=0
  wires:
  Delay14/1 -> out0/1
  in0/1 -> Delay14/1

== system gm_uz_ssi_interface_2023a/uz_ssi_interface/position_to_speed_pll/Delay18 ==
  in0 : Inport  OutDataTypeStr=fixdt(1, 27, 20)  PortDimensions=[2]  SampleTime=1e-08
  Trigger_emulated : EnablePort  OutDataTypeStr=boolean
  Delay18 : Delay  DelayLength=double(1)  InitialCondition=[1 0]
  out0 : Outport  OutDataTypeStr=fixdt(1, 27, 20)  PortDimensions=[2]  SampleTime=1e-08  InitialOutput=0
  wires:
  Delay18/1 -> out0/1
  in0/1 -> Delay18/1

== system gm_uz_ssi_interface_2023a/uz_ssi_interface/position_to_speed_pll/Delay19 ==
  in0 : Inport  OutDataTypeStr=fixdt(1, 27, 23)  SampleTime=1e-08
  Trigger_emulated : EnablePort  OutDataTypeStr=boolean
  Delay19 : Delay  DelayLength=double(1)  InitialCondition=0
  out0 : Outport  OutDataTypeStr=fixdt(1, 27, 23)  SampleTime=1e-08  InitialOutput=0
  wires:
  Delay19/1 -> out0/1
  in0/1 -> Delay19/1

== system gm_uz_ssi_interface_2023a/uz_ssi_interface/position_to_speed_pll/Delay2 ==
  in0 : Inport  OutDataTypeStr=fixdt(1, 27, 24)  SampleTime=1e-08
  Trigger_emulated : EnablePort  OutDataTypeStr=boolean
  Delay2 : Delay  DelayLength=double(1)  InitialCondition=0
  out0 : Outport  OutDataTypeStr=fixdt(1, 27, 24)  SampleTime=1e-08  InitialOutput=0
  wires:
  Delay2/1 -> out0/1
  in0/1 -> Delay2/1

== system gm_uz_ssi_interface_2023a/uz_ssi_interface/position_to_speed_pll/Delay20 ==
  in0 : Inport  OutDataTypeStr=boolean  SampleTime=1e-08
  Trigger_emulated : EnablePort  OutDataTypeStr=boolean
  Delay20 : Delay  DelayLength=double(1)  InitialCondition=0
  out0 : Outport  OutDataTypeStr=boolean  SampleTime=1e-08  InitialOutput=0
  wires:
  Delay20/1 -> out0/1
  in0/1 -> Delay20/1

== system gm_uz_ssi_interface_2023a/uz_ssi_interface/position_to_speed_pll/Delay21 ==
  in0 : Inport  OutDataTypeStr=boolean  SampleTime=1e-08
  Trigger_emulated : EnablePort  OutDataTypeStr=boolean
  Delay21 : Delay  DelayLength=double(1)  InitialCondition=0
  out0 : Outport  OutDataTypeStr=boolean  SampleTime=1e-08  InitialOutput=0
  wires:
  Delay21/1 -> out0/1
  in0/1 -> Delay21/1

== system gm_uz_ssi_interface_2023a/uz_ssi_interface/position_to_speed_pll/Delay22 ==
  in0 : Inport  OutDataTypeStr=fixdt(1, 27, 20)  SampleTime=1e-08
  Trigger_emulated : EnablePort  OutDataTypeStr=boolean
  Delay22 : Delay  DelayLength=double(1)  InitialCondition=0
  out0 : Outport  OutDataTypeStr=fixdt(1, 27, 20)  SampleTime=1e-08  InitialOutput=0
  wires:
  Delay22/1 -> out0/1
  in0/1 -> Delay22/1

== system gm_uz_ssi_interface_2023a/uz_ssi_interface/position_to_speed_pll/Delay23 ==
  in0 : Inport  OutDataTypeStr=fixdt(1, 27, 20)  SampleTime=1e-08
  Trigger_emulated : EnablePort  OutDataTypeStr=boolean
  Delay23 : Delay  DelayLength=double(1)  InitialCondition=0
  out0 : Outport  OutDataTypeStr=fixdt(1, 27, 20)  SampleTime=1e-08  InitialOutput=0
  wires:
  Delay23/1 -> out0/1
  in0/1 -> Delay23/1

== system gm_uz_ssi_interface_2023a/uz_ssi_interface/position_to_speed_pll/Delay3 ==
  in0 : Inport  OutDataTypeStr=fixdt(1, 27, 14)  SampleTime=1e-08
  Trigger_emulated : EnablePort  OutDataTypeStr=boolean
  Delay3 : Delay  DelayLength=double(1)  InitialCondition=0
  out0 : Outport  OutDataTypeStr=fixdt(1, 27, 14)  SampleTime=1e-08  InitialOutput=0
  wires:
  Delay3/1 -> out0/1
  in0/1 -> Delay3/1

== system gm_uz_ssi_interface_2023a/uz_ssi_interface/position_to_speed_pll/Delay4 ==
  in0 : Inport  OutDataTypeStr=fixdt(1, 27, 20)  SampleTime=1e-08
  Trigger_emulated : EnablePort  OutDataTypeStr=boolean
  Delay4 : Delay  DelayLength=double(1)  InitialCondition=0
  out0 : Outport  OutDataTypeStr=fixdt(1, 27, 20)  SampleTime=1e-08  InitialOutput=0
  wires:
  Delay4/1 -> out0/1
  in0/1 -> Delay4/1

== system gm_uz_ssi_interface_2023a/uz_ssi_interface/position_to_speed_pll/Delay5 ==
  in0 : Inport  OutDataTypeStr=fixdt(1, 27, 8)  SampleTime=1e-08
  Trigger_emulated : EnablePort  OutDataTypeStr=boolean
  Delay5 : Delay  DelayLength=double(1)  InitialCondition=0
  out0 : Outport  OutDataTypeStr=fixdt(1, 27, 8)  SampleTime=1e-08  InitialOutput=0
  wires:
  Delay5/1 -> out0/1
  in0/1 -> Delay5/1

== system gm_uz_ssi_interface_2023a/uz_ssi_interface/position_to_speed_pll/Delay6 ==
  in0 : Inport  OutDataTypeStr=fixdt(0, 18, 24)  SampleTime=1e-08
  Trigger_emulated : EnablePort  OutDataTypeStr=boolean
  Delay6 : Delay  DelayLength=double(1)  InitialCondition=0
  out0 : Outport  OutDataTypeStr=fixdt(0, 18, 24)  SampleTime=1e-08  InitialOutput=0
  wires:
  Delay6/1 -> out0/1
  in0/1 -> Delay6/1

== system gm_uz_ssi_interface_2023a/uz_ssi_interface/position_to_speed_pll/Delay7 ==
  in0 : Inport  OutDataTypeStr=fixdt(0, 18, 0)  SampleTime=1e-08
  Trigger_emulated : EnablePort  OutDataTypeStr=boolean
  Delay7 : Delay  DelayLength=double(1)  InitialCondition=0
  out0 : Outport  OutDataTypeStr=fixdt(0, 18, 0)  SampleTime=1e-08  InitialOutput=0
  wires:
  Delay7/1 -> out0/1
  in0/1 -> Delay7/1

== system gm_uz_ssi_interface_2023a/uz_ssi_interface/position_to_speed_pll/Delay8 ==
  in0 : Inport  OutDataTypeStr=fixdt(0, 18, 5)  SampleTime=1e-08
  Trigger_emulated : EnablePort  OutDataTypeStr=boolean
  Delay8 : Delay  DelayLength=double(1)  InitialCondition=0
  out0 : Outport  OutDataTypeStr=fixdt(0, 18, 5)  SampleTime=1e-08  InitialOutput=0
  wires:
  Delay8/1 -> out0/1
  in0/1 -> Delay8/1

== system gm_uz_ssi_interface_2023a/uz_ssi_interface/position_to_speed_pll/Delay9 ==
  in0 : Inport  OutDataTypeStr=fixdt(1, 27, 14)  SampleTime=1e-08
  Trigger_emulated : EnablePort  OutDataTypeStr=boolean
  Delay9 : Delay  DelayLength=double(1)  InitialCondition=0
  out0 : Outport  OutDataTypeStr=fixdt(1, 27, 14)  SampleTime=1e-08  InitialOutput=0
  wires:
  Delay9/1 -> out0/1
  in0/1 -> Delay9/1

== system gm_uz_ssi_interface_2023a/uz_ssi_interface/position_to_speed_pll/Sine HDL Optimized ==
  u : Inport  OutDataTypeStr=fixdt(1, 27, 20)  SampleTime=1e-08
  sincos hdl : Subsystem  mask{NumDataPoints=256, TableDataTypeStr=fixdt(0,26,20), SimulateLUTROMDelay='Off'}
      mask prompts: NumDataPoints "HDLShared:hdlshared:CosineHDL_Npts"; TableDataTypeStr "Simulink:blkprm_prompts:TABLE_UNIFIEDDATATYPE"; SimulateLUTROMDelay "HDLShared:hdlshared:CosineHDL_SimulateLUTDelay"
      mask Display:
      | port_label('input',1,'u')
      | port_label('output',1,'sin(2*pi*u)')
      | port_label('output',2,'cos(2*pi*u)')
      | xpos = 0.35;
      | yoffset = 0.5;
      | if ( SimulateLUTROMDelay )
      |   text(xpos,yoffset,'HDL (Z^{-1})','texmode','on')
      | else
      |    text(xpos,yoffset,'HDL')
      | end
  x : Outport  SampleTime=1e-08  InitialOutput=0
  y : Outport  Port=2  SampleTime=1e-08  InitialOutput=0
  wires:
  sincos hdl/1(Out1) -> x/1
  sincos hdl/2(Out2) -> y/1
  u/1 -> sincos hdl/1(In1)

== system gm_uz_ssi_interface_2023a/uz_ssi_interface/position_to_speed_pll/Sine HDL Optimized1 ==
  u : Inport  OutDataTypeStr=fixdt(1, 27, 20)  SampleTime=1e-08
  sincos hdl : Subsystem  mask{NumDataPoints=256, TableDataTypeStr=fixdt(0,26,20), SimulateLUTROMDelay='Off'}
      mask prompts: NumDataPoints "HDLShared:hdlshared:CosineHDL_Npts"; TableDataTypeStr "Simulink:blkprm_prompts:TABLE_UNIFIEDDATATYPE"; SimulateLUTROMDelay "HDLShared:hdlshared:CosineHDL_SimulateLUTDelay"
      mask Display:
      | port_label('input',1,'u')
      | port_label('output',1,'sin(2*pi*u)')
      | port_label('output',2,'cos(2*pi*u)')
      | xpos = 0.35;
      | yoffset = 0.5;
      | if ( SimulateLUTROMDelay )
      |   text(xpos,yoffset,'HDL (Z^{-1})','texmode','on')
      | else
      |    text(xpos,yoffset,'HDL')
      | end
  x : Outport  SampleTime=1e-08  InitialOutput=0
  y : Outport  Port=2  SampleTime=1e-08  InitialOutput=0
  wires:
  sincos hdl/1(Out1) -> x/1
  sincos hdl/2(Out2) -> y/1
  u/1 -> sincos hdl/1(In1)

== system gm_uz_ssi_interface_2023a/uz_ssi_interface/position_to_speed_pll/fixed_point_floor ==
  x : Inport  OutDataTypeStr=fixdt(1, 27, 23)  PortDimensions=1  SampleTime=1e-08
  fixed_point_floor : MATLAB Function  TreatAsAtomicUnit=on
  y : Outport  SampleTime=1e-08  InitialOutput=0  VectorParamsAs1DForOutWhenUnconnected=off
  wires:
  fixed_point_floor/1(y) -> y/1
  x/1 -> fixed_point_floor/1(x)

== system gm_uz_ssi_interface_2023a/uz_ssi_interface/ssi_communication/clk_idle_and_delay_first_clock_function ==
  delay_first_clk_on_off : Inport  OutDataTypeStr=boolean  PortDimensions=1  SampleTime=1e-08
  trigger_ssi : Inport  Port=2  OutDataTypeStr=boolean  PortDimensions=1  SampleTime=1e-08
  ssi_clk_enb_out : Inport  Port=3  OutDataTypeStr=boolean  PortDimensions=1  SampleTime=1e-08
  Constant4 : Constant  Value=0  OutDataTypeStr=boolean  SampleTime=1e-08
  Constant5 : Constant  OutDataTypeStr=boolean  SampleTime=1e-08
  Delay : Delay  DelayLength=double(108)  InitialCondition=0  SampleTime=1e-08
  Delay5 : Delay  DelayLength=double(1)  InitialCondition=0  SampleTime=1e-08
  Detect Rise Positive2 : simulink/Logic and Bit Operations/Detect Rise Positive  vinit=0  OutDataTypeStr=boolean
  NOT : Logic  Operator=NOT  Inputs=1  AllPortsSameDT=off  OutDataTypeStr=boolean  SampleTime=1e-08
  S-R Flip-Flop : simulink_extras/Flip Flops/S-R Flip-Flop  initial_condition=0
  S-R Flip-Flop_inst_term1 : Terminator
  Switch : Switch  Criteria=u2 > Threshold  Threshold=double(0)  OutDataTypeStr=boolean  SampleTime=1e-08  SaturateOnIntegerOverflow=off  InputSameDT=off
  Switch3 : Switch  Criteria=u2 > Threshold  Threshold=double(0)  OutDataTypeStr=boolean  SampleTime=1e-08  SaturateOnIntegerOverflow=off  InputSameDT=off
  Switch4 : Switch  Criteria=u2 > Threshold  Threshold=double(0)  OutDataTypeStr=boolean  SampleTime=1e-08  SaturateOnIntegerOverflow=off  InputSameDT=off
  ssi_clk_enb : Outport  SampleTime=1e-08
  ssi_clk_idle_levels : Outport  Port=2  SampleTime=1e-08
  wires:
  Constant4/1 -> Switch/1
  Constant5/1 -> Switch/3
  Delay/1 -> Switch4/1
  Delay5/1 -> Switch4/3, Switch4/2, Switch3/3
  Detect Rise Positive2/1 -> S-R Flip-Flop/2
  NOT/1 -> Detect Rise Positive2/1
  S-R Flip-Flop/1 -> Switch/2, Delay5/1, Delay/1
  S-R Flip-Flop/2 -> S-R Flip-Flop_inst_term1/1
  Switch/1 -> ssi_clk_idle_levels/1
  Switch3/1 -> ssi_clk_enb/1
  Switch4/1 -> Switch3/1
  delay_first_clk_on_off/1 -> Switch3/2
  trigger_ssi/1 -> S-R Flip-Flop/1
  ssi_clk_enb_out/1 -> NOT/1
